simulink model "lon_noInput"  (R2016a)
settings: Solver=VariableStepAuto  StartTime=0.0  StopTime=1000  RelTol=1e-3
undefined symbols (not defined in the file): Alon, Blon, Clon, Dlon
settings Model: Creator=Gray  LastModifiedBy=Gray

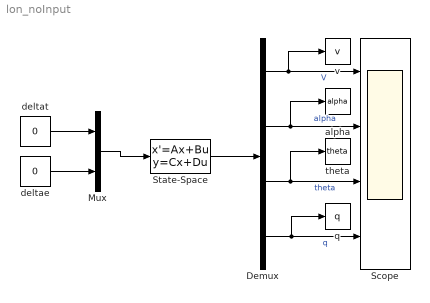
== system lon_noInput ==
  Demux : Demux
  Mux : Mux  Inputs=2
  Scope : Scope  NumInputPorts=4
  State-Space : StateSpace  A=Alon  B=Blon  C=Clon  D=Dlon  X0="[0   5/57.3 0 0]'"
  alpha : ToWorkspace  VariableName=alpha  SaveFormat=Timeseries  SampleTime=-1
  deltae : Constant  Value=0
  deltat : Constant  Value=0
  q : ToWorkspace  VariableName=q  SaveFormat=Timeseries  SampleTime=-1
  theta : ToWorkspace  VariableName=theta  SaveFormat=Timeseries  SampleTime=-1
  "v " : ToWorkspace  VariableName=v  SaveFormat=Timeseries  SampleTime=-1
  wires:
  State-Space/1 -> Demux/1
  Mux/1 -> State-Space/1
  deltat/1 -> Mux/1
  deltae/1 -> Mux/2
  Demux/1 -> "v "/1, Scope/1  "V"
  Demux/2 -> alpha/1, Scope/2  "alpha"
  Demux/3 -> theta/1, Scope/3  "theta"
  Demux/4 -> q/1, Scope/4  "q"
